simulink model "ni_e_test"  (Simulink 4.00)
settings: Solver=FixedStepDiscrete  SolverMode=SingleTasking  StartTime=0.0  StopTime=10.0  RelTol=1e-3
libraries: ni_e x8
settings Model: Creator=root  LastModifiedBy=root  SaveTime=off  SaveOutput=off  MaxDataPoints=20000  SimulationMode=external  RTWSystemTargetFile=grt_rtai.tlc  RTWOptions="-aBasePriority=30 -aExtMode=1 -aForceParamTrailComments=0 -aInlineInvariantSignals=0 -aInlineParameters=0 -aLocalBlockOutputs=1 -aLogVarNameModifier=\"rt_\" -aMatFileLogging=0 -aRTWVerbose=1 -aRollThreshold=5 -aShowEliminatedStatements=1 -aTaskStackSize=16384"  RTWTemplateMakefile=grt_rtai.tmf  ExtModeTrigDuration=10000  BlockReductionOpt=off

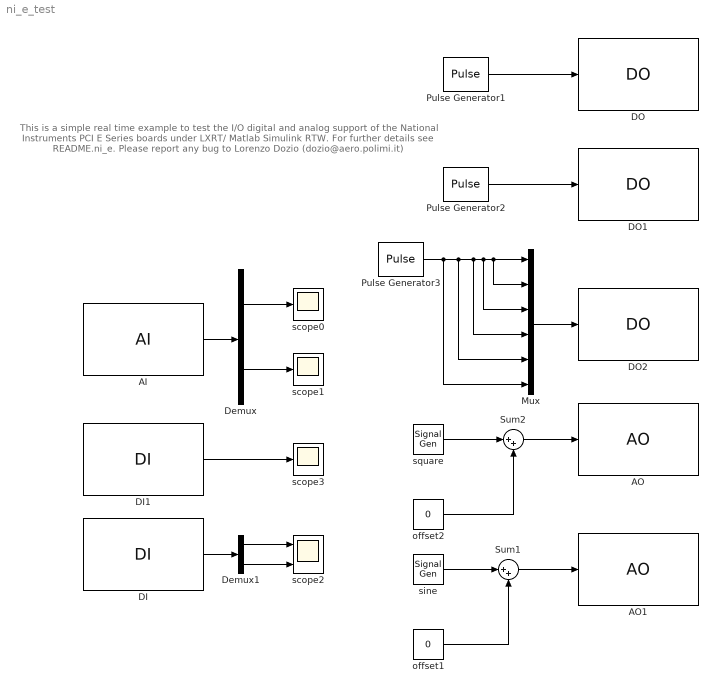
== system ni_e_test ==
  note: This is a simple real time example to test the
      | I/O digital and analog support
      | of the National Instruments PCI E Series boards
      | under LXRT/ Matlab Simulink RTW.
      | For further details see README.ni_e.
      |
      | Please report any bug to Lorenzo Dozio
      | (dozio@aero.polimi.it)
  AI : ni_e/AI  nch=2  type=RSE  gain=1  pol=bipolar  dither=off  timer=on  dt=0.0001
  AO : ni_e/AO  chan=DAC0  ref=internal  pol=bipolar  timer=on  dt=0.0001
  AO1 : ni_e/AO  chan=DAC1  ref=internal  pol=bipolar  timer=on  dt=0.0001
  DI : ni_e/DI  has_8255=on  port=A  nch_8255=2  daqstc_dio=off  nch_daqstc=1  dt=0.0001
  DI1 : ni_e/DI  has_8255=off  port=A  nch_8255=2  daqstc_dio=on  nch_daqstc=2  dt=0.0001
  DO : ni_e/DO  has_8255=off  port=B  nch_8255=4  daqstc_dio=on  nch_daqstc=1  dt=0.0001
  DO1 : ni_e/DO  has_8255=off  port=B  nch_8255=1  daqstc_dio=on  nch_daqstc=7  dt=0.0001
  DO2 : ni_e/DO  has_8255=on  port=B  nch_8255=6  daqstc_dio=off  nch_daqstc=7  dt=0.0001
  Demux : Demux  Outputs=2  BusSelectionMode=off
  Demux1 : Demux  Outputs=2  BusSelectionMode=off
  Mux : Mux  Inputs=6
  Pulse Generator1 : DiscretePulseGenerator  Amplitude=0.5  Period=50  PulseWidth=10  PhaseDelay=0  SampleTime=0.0001
  Pulse Generator2 : DiscretePulseGenerator  Amplitude=0.5  Period=50  PulseWidth=40  PhaseDelay=0  SampleTime=0.0001
  Pulse Generator3 : DiscretePulseGenerator  Amplitude=0.5  Period=50  PulseWidth=25  PhaseDelay=0  SampleTime=0.0001
  Sum1 : Sum  Inputs=|++  SaturateOnIntegerOverflow=on
  Sum2 : Sum  Inputs=|++  SaturateOnIntegerOverflow=on
  offset1 : Constant  Value=0
  offset2 : Constant  Value=0
  scope0 : Scope
      settings: TimeRange=1  YMin=-10  YMax=10  SaveToWorkspace=off  SaveName=ScopeData  MaxDataPoints=5000  SampleTime=0.0001
  scope1 : Scope
      settings: TimeRange=0.04  YMin=-10  YMax=10  SaveToWorkspace=off  LimitDataPoints=on  MaxDataPoints=200000  SampleTime=0.00005
  scope2 : Scope  NumInputPorts=2
      settings: TimeRange=0.01  YMin=-1~-1  YMax=2~2  SaveToWorkspace=off  SaveName=ScopeData2  MaxDataPoints=5000  SampleTime=0.0001
  scope3 : Scope
      settings: TimeRange=0.04  YMin=-1  YMax=2  SaveToWorkspace=off  SaveName=ScopeData3  LimitDataPoints=on  MaxDataPoints=200000  SampleTime=0.00005
  sine : SignalGenerator  WaveForm=sine  Amplitude=5  Frequency=50  Units=Hertz
  square : SignalGenerator  WaveForm=square  Amplitude=2  Frequency=30  Units=Hertz
  wires:
  offset1/1 -> Sum1/2
  Sum1/1 -> AO1/1
  sine/1 -> Sum1/1
  Demux/1 -> scope0/1
  Demux/2 -> scope1/1
  AI/1 -> Demux/1
  offset2/1 -> Sum2/2
  square/1 -> Sum2/1
  Sum2/1 -> AO/1
  Pulse Generator1/1 -> DO/1
  Pulse Generator2/1 -> DO1/1
  Pulse Generator3/1 -> Mux/1, Mux/2, Mux/3, Mux/4, Mux/5, Mux/6
  Mux/1 -> DO2/1
  DI/1 -> Demux1/1
  Demux1/1 -> scope2/1
  Demux1/2 -> scope2/2
  DI1/1 -> scope3/1
